simulink model "Assembled_descramble"  (R2024b)
settings: Solver=FixedStepAuto  StartTime=0.0  StopTime=10.0  RelTol=1e-3
undefined symbols (not defined in the file): Radix
libraries: androiduilib x3, dspxfrm3 x2, androidaudiovideolib x1, androidcommunicationlib x1, dspsigops x1
settings Model: Creator=hrida  LastModifiedBy=hrida
settings OptimizationCC: DefaultParameterBehavior=Inlined  EnhancedBackFolding=on  PassReuseOutputArgsAs=Individual arguments  ZeroExternalMemoryAtStartup=off  ZeroInternalMemoryAtStartup=off  MaxStackSize=64  OptimizeBlockOrder=speed  DifferentSizesBufferReuse=on  OptimizationCustomize=off  EfficientTunableParamExpr=on
settings DebuggingCC: ParameterTunabilityLossMsg=error
settings HardwareCC: ProdBitPerLong=64  ProdLargestAtomicInteger=LongLong  ProdLargestAtomicFloat=Double  ProdLongLongMode=on  ProdHWDeviceType=ARM Compatible->ARM Cortex-A (64-bit)
settings RTWCC: Description=Embedded Coder  SystemTargetFile=ert.tlc  HardwareBoard=Android Device (64bit)  TLCOptions="-aInlineSetEventsForThisBaseRateFcn=TLC_FALSE -aSuppressMultiTaskScheduler=TLC_FALSE  -aRateBasedStepFcn=0"  TemplateMakefile=ert_default_tmf  RTWVerbose=off  Toolchain=Android SDK/NDK Tools
settings CodeAppCC: ForceParamTrailComments=on  IgnoreCustomStorageClasses=off  OperatorAnnotations=on  SimulinkDataObjDesc=on  SFDataObjDesc=on  InsertBlockDesc=on
settings ERTTargetCC: SupportVariableSizeSignals=on

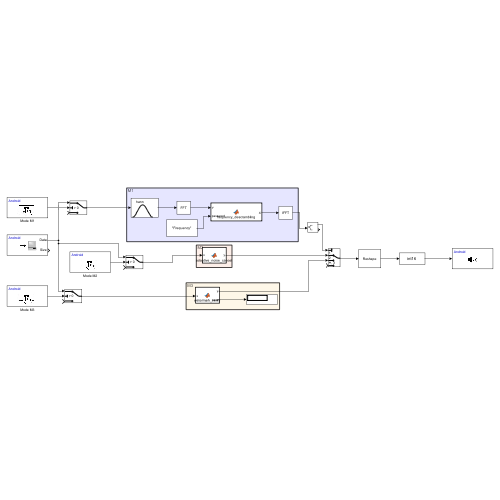
[thumbnail: Simulink's stored preview of the top-level diagram]
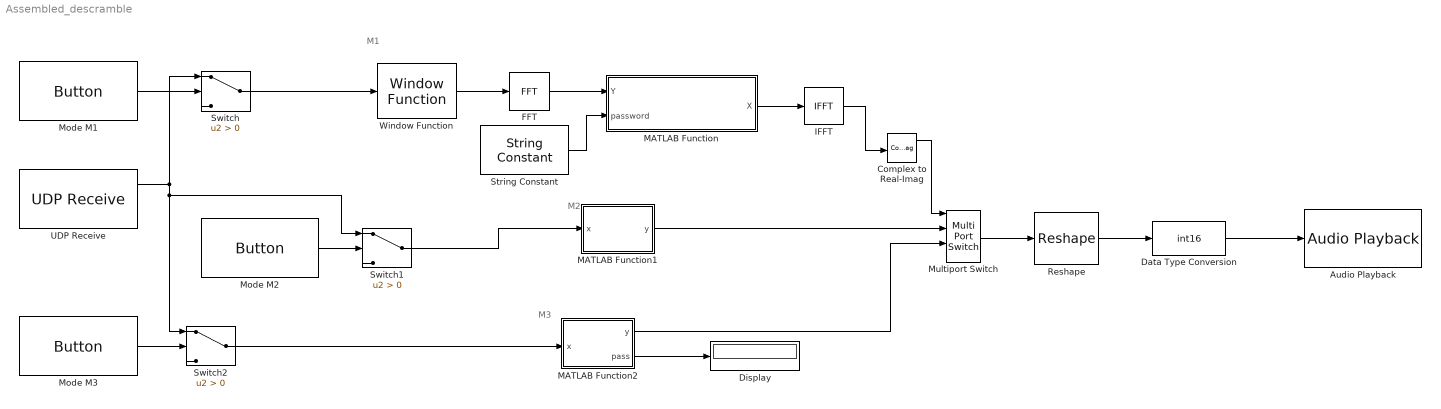
== system Assembled_descramble ==
  note: M3
  note: M2
  note: M1
  Audio Playback : androidaudiovideolib/Audio Playback  SampleFreq=16000  AudioSamplingFreq=16000  SampleTime=0.1  DeviceStr=0  QueueDuration=0  BlockPlatform=Android
  Complex to Real-Imag : ComplexToRealImag
  Data Type Conversion : DataTypeConversion  OutDataTypeStr=int16  SaturateOnIntegerOverflow=off  RndMeth=Floor
  Display : Display
  FFT : dspxfrm3/FFT  FFTImplementation=Radix-2  CompMethod=Table lookup  TableOpt=NEW  TableOptActive=Speed  BitRevOrder=off  Normalize=off  InheritFFTLength=on  FFTLength=64  WrapInput=on  roundingMode=Ceiling  overflowMode=off  firstCoeffDataTypeStr=Inherit: Same word length as input  firstCoeffLastDataTypeStr=Inherit: Same word length as input  outputMin=[]  outputMax=[]
  IFFT : dspxfrm3/IFFT  FFTImplementation=Radix-2  CompMethod=Table lookup  TableOpt=NEW  TableOptActive=Speed  BitRevOrder=off  cs_in=off  Normalize=on  InheritFFTLength=on  FFTLength=64  WrapInput=on  mode=Real  outSamplingMode=Sample based  roundingMode=Ceiling  overflowMode=off  firstCoeffDataTypeStr=Inherit: Same word length as input  firstCoeffLastDataTypeStr=Inherit: Same word length as input  accumDataTypeStr=Inherit: Same as product output  accumLastDataTypeStr=Inherit: Same as product output  outputMin=[]  outputMax=[]
  MATLAB Function : MATLAB Function  TreatAsAtomicUnit=on
  MATLAB Function1 : MATLAB Function  TreatAsAtomicUnit=on
  MATLAB Function2 : MATLAB Function  TreatAsAtomicUnit=on
  Mode M1 : androiduilib/Button  ButtonState=Not pressed  ButtonId=Assembled_descramble/Mode_M1  State=off  SampleTime=0.1  BlockPlatform=Android
  Mode M2 : androiduilib/Button  ButtonState=Not pressed  ButtonId=Assembled_descramble/Mode_M2  State=off  SampleTime=0.1  BlockPlatform=Android
  Mode M3 : androiduilib/Button  ButtonState=Not pressed  ButtonId=Assembled_descramble/Mode_M3  State=off  SampleTime=0.1  BlockPlatform=Android
  Multiport Switch : MultiPortSwitch  DiagnosticForDefault=None  SaturateOnIntegerOverflow=off  InputSameDT=off
  Reshape : Reshape  OutputDimensionality=Customize  OutputDimensions=[64,2]
  String Constant : StringConstant  String="\"Frequency\""
  Switch : Switch  Criteria=u2 > Threshold  SaturateOnIntegerOverflow=off  InputSameDT=off
  Switch1 : Switch  Criteria=u2 > Threshold  SaturateOnIntegerOverflow=off  InputSameDT=off
  Switch2 : Switch  Criteria=u2 > Threshold  SaturateOnIntegerOverflow=off  InputSameDT=off
  UDP Receive : androidcommunicationlib/UDP Receive  localURL='0.0.0.0'  localPort=25000  remoteURL='0.0.0.0'  remotePort=-1  recvBufferSize=8192  signalDatatype=double  dims=128  isVarSize=off  showBlockingTime=off  blockingTime=0  sampletime=0.064  blockPlatform=Android
  Window Function : dspsigops/Window Function  winmode=Apply window to input  wintype=Hann  sampmode=Continuous  samptime=1  N=64  Rs=50  beta=10  winsamp=Symmetric  UserWindow=hamming  OptParams=off  UserParams={'symmetric'}  dataType=double  isSigned=on  wordLen=16  udDataType=sfix(16)  fracBitsMode=Best precision  numFracBits=15  roundingMode=Floor  overflowMode=off  numSidelobes=4  sidelobeLevel=-30
  wires:
  Window Function/1 -> FFT/1
  FFT/1 -> MATLAB Function/1(Y)
  MATLAB Function1/1(y) -> Multiport Switch/2
  MATLAB Function/1(X) -> IFFT/1
  String Constant/1 -> MATLAB Function/2(password)
  MATLAB Function2/1(y) -> Multiport Switch/3
  MATLAB Function2/2(pass) -> Display/1
  Multiport Switch/1 -> Reshape/1
  UDP Receive/1 -> Switch2/1, Switch1/1, Switch/1
  Mode M1/1 -> Switch/2
  Switch/1 -> Window Function/1
  Mode M2/1 -> Switch1/2
  Switch1/1 -> MATLAB Function1/1(x)
  Mode M3/1 -> Switch2/2
  Switch2/1 -> MATLAB Function2/1(x)
  IFFT/1 -> Complex to Real-Imag/1
  Complex to Real-Imag/1 -> Multiport Switch/1
  Reshape/1 -> Data Type Conversion/1
  Data Type Conversion/1 -> Audio Playback/1

== matlab function Assembled_descramble/MATLAB Function ==
  data: Y input; X output; password input
function X = frequency_descrambling(Y,password)

    N = length(Y);          % FFT size (should be 1024)
    halfN = N/2;            % 512

    % Key regeneration
    seed = sum(double(char(password))) + length(password);
    rng(seed);
    key = randperm(halfN-1) + 1;   % indices 2..512

    % Inverse permutation (size = halfN)
    inv_key = zeros(1, halfN);
    inv_key(key) = 2:halfN;

    % Allocate output as complex
    X = complex(zeros(size(Y)));

    % Preserve DC & Nyquist
    X(1) = Y(1);
    X(halfN+1) = Y(halfN+1);

    % Apply inverse permutation
    X(2:halfN) = Y(inv_key(2:halfN));

    % Restore symmetry
    X(halfN+2:N) = conj(flipud(X(2:halfN)));

end

== matlab function Assembled_descramble/MATLAB Function2 ==
  data: x input; y output; pass output
function [y, pass] = watermark_verify(x)
fs = 16000;
N = length(x);
t = (0:N-1)/fs;
rng(12345);
wm = 0.001 * sin(2*pi*3000*t + rand(1,N));
corr_val = corrcoef(x, wm');
pass = corr_val(1,2) > 0.8; % threshold
y = x; % same audio (authentication only)
end

== matlab function Assembled_descramble/MATLAB Function1 ==
  data: x input; y output
function y = adaptive_noise_cancel(x)
N = length(x);
X = fft(x);
mag = abs(X);
NoiseEstimate = 0.1 * mag; % same shaping factor used earlier
Y = X - NoiseEstimate .* exp(1j*angle(X));
y = real(ifft(Y));
end
